simulink model "MotorImplementation"  (R2022a)
settings: Solver=FixedStepAuto  StartTime=0.0  StopTime=60  FixedStep=1/25  RelTol=1e-3
model workspace (MATLAB code in the model file):
  | %% Mechanical Parameters
  | d_Drum = 23.23e-2; % Meter
  | Drum_Friction = 0.001; % Ns/m
  | Drum_Inertia = 1.0; %kgm^2
  | 
  | n_sh = 5;
  | 
  | %% Load Case 1
  | Hs = 2.2; % m
  | T_w = 8.0; % s
  | m_payload = 8000; % kg
  | h_payload_0 = 75; % m
  | h_payload_final = h_payload_0; % m
  | h_seabed = 350; % m
  | 
  | %% Load Case 2
  | Hs = 2.2; % m
  | T_w = 8.0; % s
  | m_payload = 8000; % kg
  | h_payload_0 = 75; % m
  | h_payload_final = 15; % m
  | h_seabed = 350; % m
  | 
  | %% Load Case 3
  | Hs = 2.2; % m
  | T_w = 8.0; % s
  | m_payload = 8000; % kg
  | h_payload_0 =15; % m
  | h_payload_final = 0; % m
  | h_seabed = 350; % m
  | 
  | %% Sensors
  | % Noise simulation
  | sigma_w = 0.5; %m/s^2 (Standard deviation of noise)
  | beta = 10000; % Positive constant [-]
  | 
  | %% Payload parameters
  | % mass already defined (8000kg)
  | Volume_pl = 2; %m^3
  | Area_pl = 1.5; %m^2
  | C_D = 1.8; %[-] Drag coefficient
  | 
  | %syms rho vel
  | %F_drag = 0.5 * rho * vel^2 * C_D * Area_pl; % Density of sea water(surface) approx 1.025 kg/m^3, velocity comes from the simulation.
  | 
  | %% Seabed
  | k_spring = 1.8e6; %N/m
  | b_damper = 6.5e5; %Ns/m
  | rho = 1.025;
  | %syms delta_x
  | %if delta_x < 0
  | %    F_sb = 0;
  | %else
  | %    F_sb = k_spring*delta_x + b_damper*vel*sqrt(delta_x);
  | %end
  | 
  | %% Bouyant force
  | % The force pushing upwards when something floats down in water. Dependend
  | % on the fluid density, volume of the object falling and gravity
  | g = 9.81;
  | %F_boy = rho * Volume_pl * g;
  | 
  | %% Mechanical Parameters
  | T_N = 579 % Nominal torque [Nm]
  | PF_N = 0.85; % Nominal power factor
  | f=50;
  | n_N = 1483; % mechanical speed [rpm]
  | P_N = 90000 % Nominal mechanical power [W]
  | U = 400; % line-to-line rms stator voltage [V]
  | eta_N = 0.947; % efficiency
  | n_p = 2; % pole pairs
  | I_N=160;
  | 
  | %% Electrical parameters
  | % T-circuit
  | Rs = 0.04264;
  | L_sl = 0.3172;
  | Lm = 5.3031;
  | L_rl = 0.3172;
  | R_R = 0.0288;
  | psi_R = 20*P_N/(sqrt(2)*pi*n_p*I_N*n_N);
  | %Inv Gamma Transform
  | Lr = 5.3031 + 0.3172;
  | L_M = 5.3031^2/Lr;
  | L_M_hat = 5;
  | 
  | PSI_R = 5.3031/Lr * psi_R;
  | L_sigma =((5.3031+0.3172) - Lr);
  | %L_sigma_hat = 0.12;
  | RR = (5.3031/Lr)^2 * 0.0288;
  | %RR_Hat = 0.025;
  | R_R_opt = 0.0193;
  | X_M_opt = 2.81;
  | X_sig_opt = 0.0445;
  | 
  | R_R_hat = 0.02;
  | X_M_hat = 3;
  | X_sig_hat = 0.05;
  | R_s = 0.04264;
  | %% Control parameters
  | omega_bw = log(9)/1e-3;
  | kp = omega_bw * X_sig_hat;
  | ki = omega_bw^2 * X_sig_hat;
undefined symbols (not defined in the file): I_max, L_sigma_hat, magnitude, omega_1_N, psi_ref, R_hat, RR_Hat, Ts, V_base, w_BW
libraries: fl_lib x22, nesl_utility x10, CustomComponents_lib x6, slpidlib x4, simulink x3, eeTransforms x2, sdl_lib x1
(part 1 of 2)
settings Model: Creator=Jakob  LastModifiedBy=Jakob
settings DebuggingCC: AlgebraicLoopMsg=none

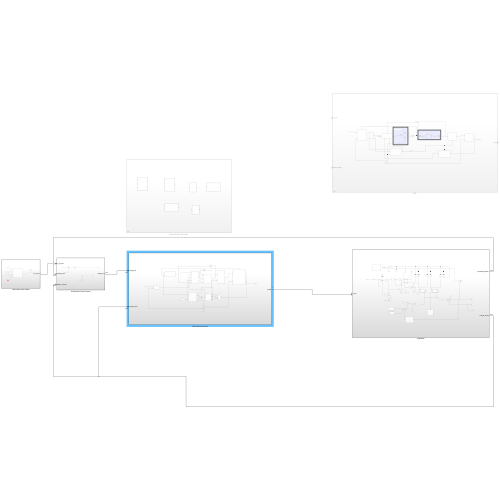
[thumbnail: Simulink's stored preview of the top-level diagram]
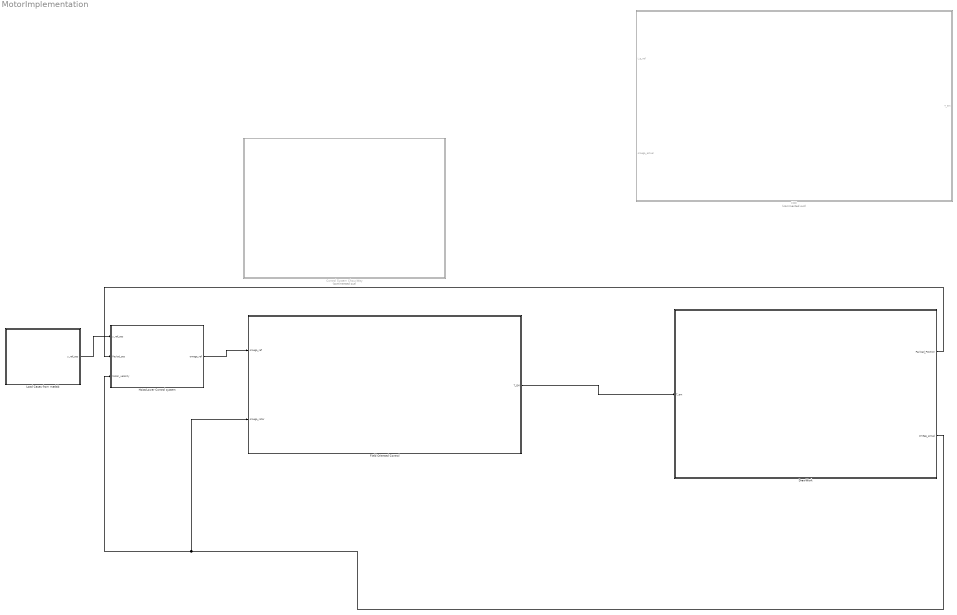
== system MotorImplementation ==
  Control System ChouxWay : Subsystem  Commented=on
  DrawWork : Subsystem
  FOC : Subsystem  Commented=on
  Field Oriented Control : Subsystem
  Hoist/Lower Control system : Subsystem
  Load Cases from matlab : Subsystem
  wires:
  Load Cases from matlab/1(y_ref_pos) -> Hoist/Lower Control system/1(y_ref_pos)
  DrawWork/1(Payload_Position) -> Hoist/Lower Control system/2(Paylod_pos)
  DrawWork/2(omega_actual) -> Field Oriented Control/2(omega_rotor), Hoist/Lower Control system/3(Motor_velocity)
  Field Oriented Control/1(T_EM) -> DrawWork/1(T_em)
  Hoist/Lower Control system/1(omega_ref) -> Field Oriented Control/1(omega_ref)

== system MotorImplementation/Control System ChouxWay ==
  Current Controller : Subsystem
  Field Weakening : Subsystem
  FluxEstimator : Subsystem
  IM Motor : Subsystem
  abc > dq : Subsystem
  "dq -> ABC" : Subsystem

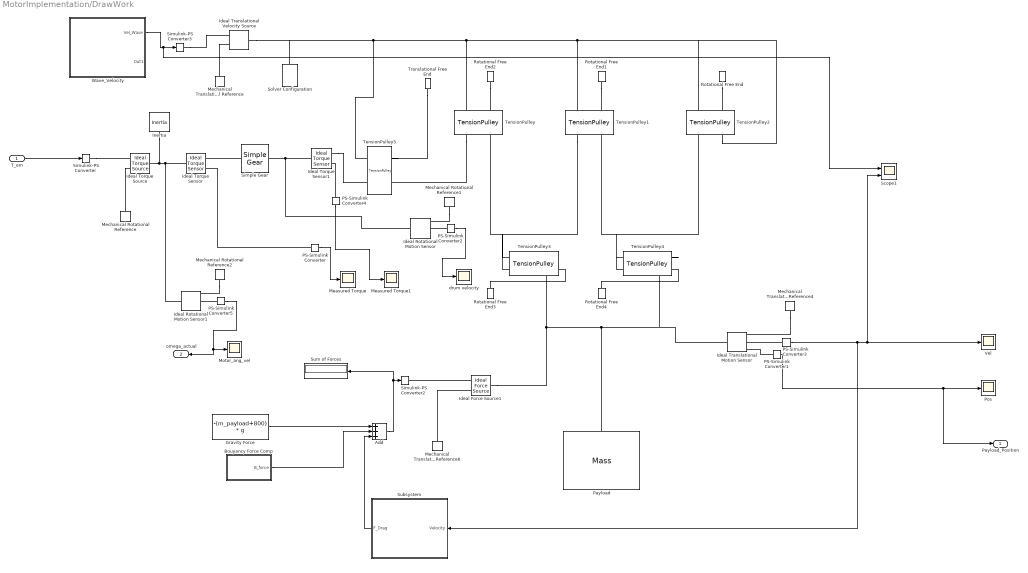
== system MotorImplementation/DrawWork ==
  T_em : Inport
  Add : Sum  Inputs=+++
  Bouyancy Force Comp : Subsystem
  Gravity Force : Constant  Value=-(m_payload+800) * g
  Ideal Force Source1 : fl_lib/Mechanical/Mechanical Sources/Ideal Force Source
      settings: SourceProductBaseCode=PW,SS,VE
  Ideal Rotational Motion Sensor : fl_lib/Mechanical/Mechanical Sensors/Ideal Rotational Motion Sensor  wrap_angle=simscape.enum.onoff.off  offset=0 rad
      settings: SourceProductBaseCode=PW,SS,VE
  Ideal Rotational Motion Sensor1 : fl_lib/Mechanical/Mechanical Sensors/Ideal Rotational Motion Sensor  wrap_angle=simscape.enum.onoff.off  offset=0 rad
      settings: SourceProductBaseCode=PW,SS,VE
  Ideal Torque Sensor : fl_lib/Mechanical/Mechanical Sensors/Ideal Torque Sensor
      settings: SourceProductBaseCode=PW,SS,VE
  Ideal Torque Sensor1 : fl_lib/Mechanical/Mechanical Sensors/Ideal Torque Sensor
      settings: SourceProductBaseCode=PW,SS,VE
  Ideal Torque Source : fl_lib/Mechanical/Mechanical Sources/Ideal Torque Source
      settings: SourceProductBaseCode=PW,SS,VE
  Ideal Translational Motion Sensor : fl_lib/Mechanical/Mechanical Sensors/Ideal Translational Motion Sensor  offset=70 m
      settings: SourceProductBaseCode=PW,SS,VE
  Ideal Translational Velocity Source : fl_lib/Mechanical/Mechanical Sources/Ideal Translational Velocity Source
      settings: SourceProductBaseCode=PW,SS,VE
  Inertia : fl_lib/Mechanical/Rotational Elements/Inertia  inertia=1.5 kg*m^2  num_ports=foundation.enum.numPorts2.one  w_specify=off  w_priority=High  w=0 rad/s  w_nominal_specify=off  w_nominal_unit=rad/s  w_nominal_value=1  t_specify=on  t_priority=None  t=500 N*m  t_nominal_specify=off  t_nominal_unit=N*m  t_nominal_value=1
      settings: SourceProductBaseCode=PW,SS,VE
  Measured Torque : Scope
  Measured Torque1 : Scope
  Mechanical Rotational Reference : fl_lib/Mechanical/Rotational Elements/Mechanical Rotational Reference
      settings: SourceProductBaseCode=PW,SS,VE
  Mechanical Rotational Reference1 : fl_lib/Mechanical/Rotational Elements/Mechanical Rotational Reference
      settings: SourceProductBaseCode=PW,SS,VE
  Mechanical Rotational Reference2 : fl_lib/Mechanical/Rotational Elements/Mechanical Rotational Reference
      settings: SourceProductBaseCode=PW,SS,VE
  Mechanical Translational Reference : fl_lib/Mechanical/Translational Elements/Mechanical Translational Reference
      settings: SourceProductBaseCode=PW,SS,VE
  Mechanical Translational Reference4 : fl_lib/Mechanical/Translational Elements/Mechanical Translational Reference
      settings: SourceProductBaseCode=PW,SS,VE
  Mechanical Translational Reference6 : fl_lib/Mechanical/Translational Elements/Mechanical Translational Reference
      settings: SourceProductBaseCode=PW,SS,VE
  Motor_ang_vel : Scope
  PS-Simulink Converter{,1..5} (6 alike) : nesl_utility/PS-Simulink Converter  PhysicalDomain=network_engine_domain  SubClassName=ps_output  LeftPortType=input  RightPortType=output  PseudoPeriodic=off  Frequencies=[]  VectorFormat=inherit  Unit=inherit  AffineConversion=off
      settings: SourceProductBaseCode=SS,PW,VE
  Payload : fl_lib/Mechanical/Translational Elements/Mass  mass=8800 kg  num_ports=foundation.enum.numPorts2.one  v_specify=off  v_priority=High  v=0 m/s  v_nominal_specify=off  v_nominal_unit=m/s  v_nominal_value=1  f_specify=off  f_priority=None  f=0 N  f_nominal_specify=off  f_nominal_unit=N  f_nominal_value=1
      settings: SourceProductBaseCode=PW,SS,VE
  Pos : Scope
  Rotational Free End{,1..4} (5 alike) : fl_lib/Mechanical/Rotational Elements/Rotational Free End  w_specify=off  w_priority=None  w=0 rad/s  w_nominal_specify=off  w_nominal_unit=rad/s  w_nominal_value=1
      settings: SourceProductBaseCode=PW,SS,VE
  Scope1 : Scope  NumInputPorts=2
  Simple Gear : sdl_lib/Gears/Simple Gear  ratio=5  rotation_direction=sdl.enum.shaftOutputDirection.opposite  friction_model=sdl.enum.gear_efficiencies_load.off  T_noload=0.1 N*m  T_nom=5 N*m  efficiency_nom=0.8  efficiency=0.8  temperature_TLU=[280, 300, 320] K  load_TLU=[1, 5, 10] N*m  efficiency_TLU=[.95, .9, .85]  efficiency_TLU2=[.85, .8, .75; .95, .9, .85; .85, .8, .7]  w_thr=0.01 rad/s  pwr_thr=0.001 W  backlash_model=sdl.enum.backlashModel.Off  backlash_distance=1e-3 mm  x0=0 mm  r_base=0.1 m  hardstop_model=simscape.enum.hardstop.smooth  transition=1e-4 mm  backlash_stiffness=1e7 N/m  backlash_damping=1e6 N*s/m  e=0  v_tol=0.001 m/s  mu_visc=[0, 0] N*m*s/rad  enable_faults=simscape.enum.onoff.off  efficiency_fault=0.05  external_fault=simscape.enum.onoff.off  temporal_fault=simscape.enum.onoff.off  fault_time=5 s  fault_angles=pi / 12 rad  report_fault=simscape.enum.assert.action.none  thermal_mass=50 J/K  temperature_specify=off  temperature_priority=High  temperature=300 K  temperature_nominal_specify=off  temperature_nominal_unit=K  temperature_nominal_value=1  x_backlash_specify=off  x_backlash_priority=None  x_backlash=0 mm  x_backlash_nominal_specify=off  x_backlash_nominal_unit=mm  x_backlash_nominal_value=1  f_hardstop_specify=off  f_hardstop_priority=None  f_hardstop=0 N  f_hardstop_nominal_specify=off  f_hardstop_nominal_unit=N  f_hardstop_nominal_value=1  v_backlash_specify=off  v_backlash_priority=None  v_backlash=0 m/s  v_backlash_nominal_specify=off  v_backlash_nominal_unit=m/s  v_backlash_nominal_value=1
  Simulink-PS Converter : nesl_utility/Simulink-PS Converter  PhysicalDomain=network_engine_domain  SubClassName=ps_input  LeftPortType=input  RightPortType=output  PseudoPeriodic=off  Frequencies=[]  NoiseDistribution=none  NoiseParameters=[]  Unit=1  AffineConversion=off  FilteringAndDerivatives=provide  SimscapeFilterOrder=1  InputFilterTimeConstant=0.001  UdotUserProvided=0
      settings: SourceProductBaseCode=SS,PW,VE
  Simulink-PS Converter2 : nesl_utility/Simulink-PS Converter  PhysicalDomain=network_engine_domain  SubClassName=ps_input  LeftPortType=input  RightPortType=output  PseudoPeriodic=off  Frequencies=[]  NoiseDistribution=none  NoiseParameters=[]  Unit=1  AffineConversion=off  FilteringAndDerivatives=provide  SimscapeFilterOrder=1  InputFilterTimeConstant=0.001  UdotUserProvided=0
      settings: SourceProductBaseCode=SS,PW,VE
  Simulink-PS Converter3 : nesl_utility/Simulink-PS Converter  PhysicalDomain=network_engine_domain  SubClassName=ps_input  LeftPortType=input  RightPortType=output  PseudoPeriodic=off  Frequencies=[]  NoiseDistribution=none  NoiseParameters=[]  Unit=1  AffineConversion=off  FilteringAndDerivatives=filter  SimscapeFilterOrder=2  InputFilterTimeConstant=0.001  UdotUserProvided=0
      settings: SourceProductBaseCode=SS,PW,VE
  Solver Configuration : nesl_utility/Solver Configuration  PhysicalDomain=network_engine_domain  SubClassName=solver  LeftPortType=input  RightPortType=generic  Tones=[]  Harmonics=[]  SimulateNoise=off  Profile=off  UseLocalSampling=off  EnableSwitchedLinearOptims=on  FrequencyDomain=off  UseCCode=off  RelTol=0.001  AbsTol=0.001  MinStep=1e-09  ToWorkspace=off  RevertToSquareIcSolve=off  NumHomotopyIterations=100  PhasorMode=off  PhasorModeNumHarmonics=1  IndexReductionMethod=DerivativeReplacement  DoDC=off  ResidualTolerance=1e-09  UseLocalSolver=off  LocalSolverChoice=NE_BACKWARD_EULER_ADVANCER  LocalSolverSampleTime=0.001  DoFixedCost=off  MaxNonlinIter=3  MaxModeIter=2  ComputeImpulses=off  ImpulseIterations=2  LinearAlgebra=auto  LinearAlgebraNumThread=0  EquationFormulation=NE_TIME_EF  DelaysMemoryBudget=1024  AutomaticFiltering=on  FilteringTimeConstant=0.001  PartitionStorageMethod=AS_NEEDED  PartitionMemoryBudget=1024  PartitionMethod=ROBUST
      settings: SourceProductBaseCode=SS,PW,VE
  Subsystem : Subsystem
  Sum of Forces : Display
  TensionPulley{,1..2,4} (4 alike) : CustomComponents_lib/TensionPulley  radius=0.1 m  b_damp=0 N*m*s/rad  inertia=0.00001 kg*m^2  mass=0.1 kg  mu_s=1  f_A_specify=off  f_A_priority=None  f_A=0 N  f_A_nominal_specify=off  f_A_nominal_unit=N  f_A_nominal_value=1  f_B_specify=off  f_B_priority=None  f_B=0 N  f_B_nominal_specify=off  f_B_nominal_unit=N  f_B_nominal_value=1  f_C_specify=off  f_C_priority=None  f_C=0 N  f_C_nominal_specify=off  f_C_nominal_unit=N  f_C_nominal_value=1  tau_specify=off  tau_priority=None  tau=0 N*m  tau_nominal_specify=off  tau_nominal_unit=N*m  tau_nominal_value=1  w_specify=off  w_priority=None  w=0 rad/s  w_nominal_specify=off  w_nominal_unit=rad/s  w_nominal_value=1  v_specify=off  v_priority=None  v=0 m/s  v_nominal_specify=off  v_nominal_unit=m/s  v_nominal_value=1
      settings: InternalSimscapePortConfiguration="{\"Bottom\":[],\"Left\":[{\"id\":\"C\",\"label\":\"C\",\"type\":\"foundation.mechanical.translational.translational\"},{\"id\":\"S\",\"label\":\"S\",\"type\":\"foundation.mechanical.rotational.rotational\"}],\"Right\":[{\"id\":\"A\",\"label\":\"A\",\"type\":\"foundation.mechanical.translational.translational\"},{\"id\":\"B\",\"label\":\"B\",\"type\":\"foundation.mechanical.translational.translational\"}],\"Top\":[]}"
  TensionPulley3 : CustomComponents_lib/TensionPulley  radius=0.1 m  b_damp=0 N*m*s/rad  inertia=00.00001 kg*m^2  mass=0.1 kg  mu_s=1  f_A_specify=off  f_A_priority=None  f_A=0 N  f_A_nominal_specify=off  f_A_nominal_unit=N  f_A_nominal_value=1  f_B_specify=off  f_B_priority=None  f_B=0 N  f_B_nominal_specify=off  f_B_nominal_unit=N  f_B_nominal_value=1  f_C_specify=off  f_C_priority=None  f_C=0 N  f_C_nominal_specify=off  f_C_nominal_unit=N  f_C_nominal_value=1  tau_specify=off  tau_priority=None  tau=0 N*m  tau_nominal_specify=off  tau_nominal_unit=N*m  tau_nominal_value=1  w_specify=off  w_priority=None  w=0 rad/s  w_nominal_specify=off  w_nominal_unit=rad/s  w_nominal_value=1  v_specify=off  v_priority=None  v=0 m/s  v_nominal_specify=off  v_nominal_unit=m/s  v_nominal_value=1
      settings: InternalSimscapePortConfiguration="{\"Bottom\":[],\"Left\":[{\"id\":\"C\",\"label\":\"C\",\"type\":\"foundation.mechanical.translational.translational\"},{\"id\":\"S\",\"label\":\"S\",\"type\":\"foundation.mechanical.rotational.rotational\"}],\"Right\":[{\"id\":\"A\",\"label\":\"A\",\"type\":\"foundation.mechanical.translational.translational\"},{\"id\":\"B\",\"label\":\"B\",\"type\":\"foundation.mechanical.translational.translational\"}],\"Top\":[]}"
  TensionPulley5 : CustomComponents_lib/TensionPulley  radius=d_Drum/2 m  b_damp=Drum_Friction N*m*s/rad  inertia=Drum_Inertia kg*m^2  mass=0.1 kg  mu_s=1  f_A_specify=off  f_A_priority=None  f_A=0 N  f_A_nominal_specify=off  f_A_nominal_unit=N  f_A_nominal_value=1  f_B_specify=off  f_B_priority=None  f_B=0 N  f_B_nominal_specify=off  f_B_nominal_unit=N  f_B_nominal_value=1  f_C_specify=off  f_C_priority=None  f_C=0 N  f_C_nominal_specify=off  f_C_nominal_unit=N  f_C_nominal_value=1  tau_specify=off  tau_priority=None  tau=0 N*m  tau_nominal_specify=off  tau_nominal_unit=N*m  tau_nominal_value=1  w_specify=off  w_priority=None  w=0 rad/s  w_nominal_specify=off  w_nominal_unit=rad/s  w_nominal_value=1  v_specify=off  v_priority=None  v=0 m/s  v_nominal_specify=off  v_nominal_unit=m/s  v_nominal_value=1
      settings: InternalSimscapePortConfiguration="{\"Bottom\":[],\"Left\":[{\"id\":\"C\",\"label\":\"C\",\"type\":\"foundation.mechanical.translational.translational\"},{\"id\":\"S\",\"label\":\"S\",\"type\":\"foundation.mechanical.rotational.rotational\"}],\"Right\":[{\"id\":\"A\",\"label\":\"A\",\"type\":\"foundation.mechanical.translational.translational\"},{\"id\":\"B\",\"label\":\"B\",\"type\":\"foundation.mechanical.translational.translational\"}],\"Top\":[]}"
  Translational Free End : fl_lib/Mechanical/Translational Elements/Translational Free End  v_specify=off  v_priority=None  v=0 m/s  v_nominal_specify=off  v_nominal_unit=m/s  v_nominal_value=1
      settings: SourceProductBaseCode=PW,SS,VE  InternalSimscapePortConfiguration="{\"Bottom\":[],\"Left\":[{\"id\":\"V\",\"label\":\"\",\"type\":\"foundation.mechanical.translational.translational\"}],\"Right\":[],\"Top\":[]}"
  Vel : Scope
  Wave_Velocity : Subsystem
  drum velocity : Scope
  Payload_Position : Outport
  omega_actual : Outport  Port=2
  wires:
  Subsystem/1(F_Drag) -> Add/3
  Bouyancy Force Comp/1(B_force) -> Add/2
  Add/1 -> Sum of Forces/1, Simulink-PS Converter2/1
  PS-Simulink Converter2/1 -> drum velocity/1
  PS-Simulink Converter/1 -> Measured Torque/1
  Wave_Velocity/1(Vel_Wave) -> Scope1/1, Simulink-PS Converter3/1
  PS-Simulink Converter3/1 -> Subsystem/1(Velocity), Scope1/2, Vel/1
  Gravity Force/1 -> Add/1
  PS-Simulink Converter1/1 -> Payload_Position/1, Pos/1
  PS-Simulink Converter4/1 -> Measured Torque1/1
  PS-Simulink Converter5/1 -> omega_actual/1, Motor_ang_vel/1
  T_em/1 -> Simulink-PS Converter/1
  connections:
  Ideal Torque Source/LConn1 -- Inertia/LConn1 -- Ideal Rotational Motion Sensor1/LConn1 -- Ideal Torque Sensor/LConn1
  TensionPulley4/LConn1 -- Ideal Translational Motion Sensor/LConn1 -- Payload/LConn1 -- TensionPulley3/LConn1 -- Ideal Force Source1/LConn1
  TensionPulley/LConn1 -- TensionPulley2/LConn1 -- TensionPulley2/RConn2 -- TensionPulley1/LConn1 -- TensionPulley5/LConn1 -- Solver Configuration/RConn1 -- Ideal Translational Velocity Source/LConn1
  Rotational Free End3/LConn1 -- TensionPulley3/LConn2
  TensionPulley4/RConn1 -- TensionPulley2/RConn1
  Simulink-PS Converter/RConn1 -- Ideal Torque Source/RConn1
  Ideal Force Source1/RConn1 -- Simulink-PS Converter2/RConn1
  Rotational Free End/LConn1 -- TensionPulley2/LConn2
  Mechanical Rotational Reference1/LConn1 -- Ideal Rotational Motion Sensor/RConn1
  Simulink-PS Converter3/RConn1 -- Ideal Translational Velocity Source/RConn1
  PS-Simulink Converter1/LConn1 -- Ideal Translational Motion Sensor/RConn3
  PS-Simulink Converter2/LConn1 -- Ideal Rotational Motion Sensor/RConn2
  Mechanical Rotational Reference/LConn1 -- Ideal Torque Source/RConn2
  Mechanical Translational Reference6/LConn1 -- Ideal Force Source1/RConn2
  Ideal Rotational Motion Sensor/LConn1 -- Simple Gear/RConn1 -- Ideal Torque Sensor1/LConn1
  Rotational Free End4/LConn1 -- TensionPulley4/LConn2
  PS-Simulink Converter3/LConn1 -- Ideal Translational Motion Sensor/RConn2
  TensionPulley3/RConn2 -- TensionPulley/RConn2
  TensionPulley4/RConn2 -- TensionPulley1/RConn2
  Mechanical Translational Reference4/LConn1 -- Ideal Translational Motion Sensor/RConn1
  PS-Simulink Converter/LConn1 -- Ideal Torque Sensor/RConn2
  Rotational Free End1/LConn1 -- TensionPulley1/LConn2
  TensionPulley1/RConn1 -- TensionPulley3/RConn1
  Mechanical Translational Reference/LConn1 -- Ideal Translational Velocity Source/RConn2
  Rotational Free End2/LConn1 -- TensionPulley/LConn2
  TensionPulley/RConn1 -- TensionPulley5/RConn2
  Translational Free End/LConn1 -- TensionPulley5/RConn1
  Ideal Torque Sensor1/RConn1 -- TensionPulley5/LConn2
  PS-Simulink Converter4/LConn1 -- Ideal Torque Sensor1/RConn2
  Simple Gear/LConn1 -- Ideal Torque Sensor/RConn1
  PS-Simulink Converter5/LConn1 -- Ideal Rotational Motion Sensor1/RConn2
  Mechanical Rotational Reference2/LConn1 -- Ideal Rotational Motion Sensor1/RConn1

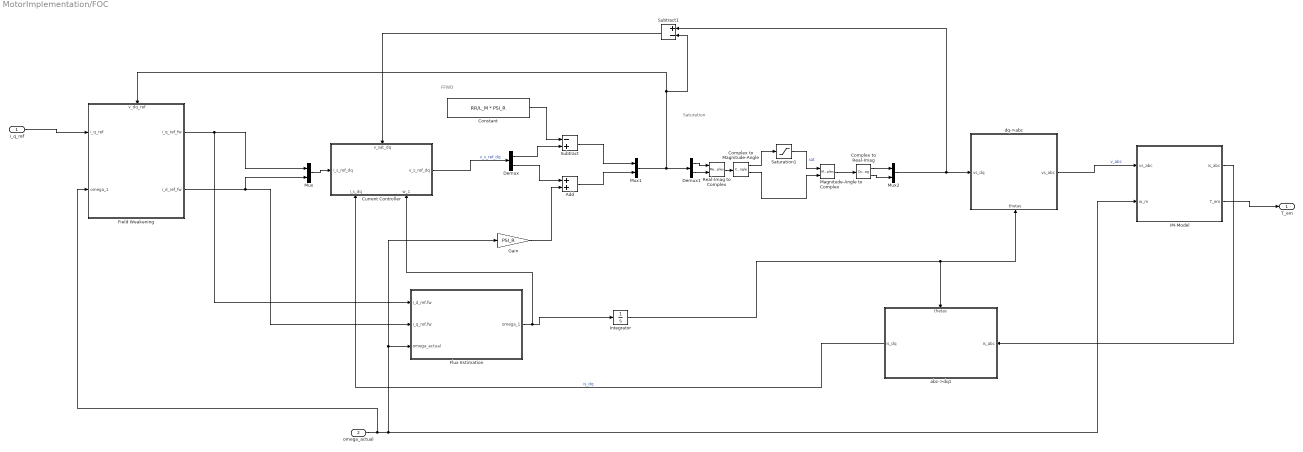
== system MotorImplementation/FOC ==
  note: Saturation
  note: FFWD
  i_q_ref : Inport
  omega_actual : Inport  Port=2
  Add : Sum
  Complex to Magnitude-Angle : ComplexToMagnitudeAngle
  Complex to Real-Imag : ComplexToRealImag
  Constant : Constant  Value=RR/L_M * PSI_R
  Current Controller : Subsystem
      settings: PortSchema="{\"entries\":[{\"content\":{\"sides\":[{\"content\":{\"connectorIds\":[\"In1\"]},\"type\":\"ConnectorPlacement.EquallySpacedRectSide\",\"uuid\":\"97c548b6-6990-4323-a853-1e64e742285c\"},{\"content\":{\"connectorIds\":[\"Out1\"],\"side\":\"RIGHT\"},\"type\":\"ConnectorPlacement.EquallySpacedRectSide\",\"uuid\":\"cacb7644-0a67-4de4-9bb2-887734fe331a\"},{\"content\":{\"connectorIds\":[\"In2\"],\"side\":\"TOP\"},\"type\":\"ConnectorPlacement.EquallySpacedRectSide\",\"uuid\":\"a20c1423-7334-426c-a525-8bdb26886bc3\"},{\"content\":{\"connectorIds\":[\"In3\",\"In4\"],\"side\":\"BOTTOM\"},\"type\":\"ConnectorPlacement.EquallySpacedRectSide\",\"uuid\":\"b9821709-22a3-4c1b-ad46-11760bdb190f\"}]},\"type\":\"ConnectorPlacement.EquallySpacedConnector\",\"uuid\":\"74caaff1-86aa-4f34-8e3a-31d84a5552f1\"}],\"packageUris\":[\"http://schema.mathworks.com/mf0/Connector/R2020b\"],\"version\":\"1.0\"}"
  Demux : Demux  Outputs=2
  Demux1 : Demux  Outputs=2
  Field Weakening : Subsystem
      settings: PortSchema="{\"entries\":[{\"content\":{\"sides\":[{\"content\":{\"connectorIds\":[\"In1\",\"In2\"]},\"type\":\"ConnectorPlacement.EquallySpacedRectSide\",\"uuid\":\"92991972-79b1-4c20-b1be-c048af0edf88\"},{\"content\":{\"connectorIds\":[\"Out1\",\"Out2\"],\"side\":\"RIGHT\"},\"type\":\"ConnectorPlacement.EquallySpacedRectSide\",\"uuid\":\"cfb4a663-faee-454f-9ec9-68645b776424\"},{\"content\":{\"connectorIds\":[\"In3\"],\"side\":\"TOP\"},\"type\":\"ConnectorPlacement.EquallySpacedRectSide\",\"uuid\":\"6b878172-644f-4a73-b905-9ff1fa4855ef\"}]},\"type\":\"ConnectorPlacement.EquallySpacedConnector\",\"uuid\":\"11cec5aa-34fb-4a6f-afd2-d847060dc809\"}],\"packageUris\":[\"http://schema.mathworks.com/mf0/Connector/R2020b\"],\"version\":\"1.0\"}"
  Flux Estimation : Subsystem
  Gain : Gain  Gain=PSI_R
  IM-Model : Subsystem
  Integrator : Integrator
  Magnitude-Angle to Complex : MagnitudeAngleToComplex
  Mux : Mux  Inputs=2
  Mux1 : Mux  Inputs=2
  Mux2 : Mux  Inputs=2
  Real-Imag to Complex : RealImagToComplex
  Saturation1 : Saturate  UpperLimit=400*sqrt(2)/sqrt(3)
  Subtract : Sum  Inputs=-+
  Subtract1 : Sum  Inputs=+-
  abc->dq1 : Subsystem
      settings: PortSchema="{\"entries\":[{\"content\":{\"sides\":[{\"content\":{\"connectorIds\":[\"In1\"]},\"type\":\"ConnectorPlacement.EquallySpacedRectSide\",\"uuid\":\"c3863cce-4a98-427c-9e63-89298f679a84\"},{\"content\":{\"connectorIds\":[\"Out1\"],\"side\":\"RIGHT\"},\"type\":\"ConnectorPlacement.EquallySpacedRectSide\",\"uuid\":\"ae3c4991-ab62-4114-9bee-e9a7348a29ce\"},{\"content\":{\"connectorIds\":[\"In2\"],\"side\":\"TOP\"},\"type\":\"ConnectorPlacement.EquallySpacedRectSide\",\"uuid\":\"fea582b6-68e0-450b-8231-0f2cf258215e\"},{\"content\":{\"connectorIds\":[],\"side\":\"BOTTOM\"},\"type\":\"ConnectorPlacement.EquallySpacedRectSide\",\"uuid\":\"4cb5cb50-d1c5-41cc-b580-d3f7a61a133b\"}]},\"type\":\"ConnectorPlacement.EquallySpacedConnector\",\"uuid\":\"936995e1-3667-4d5a-83ac-5ed23eb7cec5\"}],\"packageUris\":[\"http://schema.mathworks.com/mf0/Connector/R2020b\"],\"version\":\"1.0\"}"
  dq->abc : Subsystem
      settings: PortSchema="{\"entries\":[{\"content\":{\"sides\":[{\"content\":{\"connectorIds\":[\"In1\"]},\"type\":\"ConnectorPlacement.EquallySpacedRectSide\",\"uuid\":\"c3863cce-4a98-427c-9e63-89298f679a84\"},{\"content\":{\"connectorIds\":[\"Out1\"],\"side\":\"RIGHT\"},\"type\":\"ConnectorPlacement.EquallySpacedRectSide\",\"uuid\":\"ae3c4991-ab62-4114-9bee-e9a7348a29ce\"},{\"content\":{\"connectorIds\":[],\"side\":\"TOP\"},\"type\":\"ConnectorPlacement.EquallySpacedRectSide\",\"uuid\":\"fea582b6-68e0-450b-8231-0f2cf258215e\"},{\"content\":{\"connectorIds\":[\"In2\"],\"side\":\"BOTTOM\"},\"type\":\"ConnectorPlacement.EquallySpacedRectSide\",\"uuid\":\"09df17c4-38be-4fcd-b44b-abaf9d5b2651\"}]},\"type\":\"ConnectorPlacement.EquallySpacedConnector\",\"uuid\":\"936995e1-3667-4d5a-83ac-5ed23eb7cec5\"}],\"packageUris\":[\"http://schema.mathworks.com/mf0/Connector/R2020b\"],\"version\":\"1.0\"}"
  T_em : Outport
  wires:
  Flux Estimation/1(omega_1) -> Current Controller/4(w_1), Integrator/1
  Field Weakening/1(i_q_ref_fw) -> Mux/1, Flux Estimation/1(i_d_ref.fw)
  omega_actual/1 -> IM-Model/2(w_m), Gain/1, Flux Estimation/3(omega_actual), Field Weakening/2(omega_1)
  i_q_ref/1 -> Field Weakening/1(i_q_ref)
  Field Weakening/2(i_d_ref_fw) -> Flux Estimation/2(i_q_ref.fw), Mux/2
  Mux/1 -> Current Controller/1(i_s_ref_dq)
  Current Controller/1(v_s_ref_dq) -> Demux/1  "v_s_ref_dq"
  Gain/1 -> Add/2
  Constant/1 -> Subtract/1
  Demux/1 -> Subtract/2
  Demux/2 -> Add/1
  Subtract/1 -> Mux1/1
  Add/1 -> Mux1/2
  Demux1/2 -> Real-Imag to Complex/2
  Mux2/1 -> Subtract1/1, dq->abc/1(vs_dq)
  Saturation1/1 -> Magnitude-Angle to Complex/1  "sat"
  Complex to Real-Imag/2 -> Mux2/2
  Magnitude-Angle to Complex/1 -> Complex to Real-Imag/1
  Complex to Magnitude-Angle/2 -> Magnitude-Angle to Complex/2
  Mux1/1 -> Subtract1/2, Field Weakening/3(v_dq_ref), Demux1/1
  Real-Imag to Complex/1 -> Complex to Magnitude-Angle/1
  Complex to Magnitude-Angle/1 -> Saturation1/1
  Demux1/1 -> Real-Imag to Complex/1
  Complex to Real-Imag/1 -> Mux2/1
  dq->abc/1(vs_abc) -> IM-Model/1(vs_abc)  "v_abc"
  IM-Model/2(T_em) -> T_em/1
  IM-Model/1(is_abc) -> abc->dq1/1(is_abc)
  Integrator/1 -> abc->dq1/2(thetas), dq->abc/2(thetas)
  abc->dq1/1(is_dq) -> Current Controller/3(i_s_dq)  "is_dq"
  Subtract1/1 -> Current Controller/2(v_sat_dq)

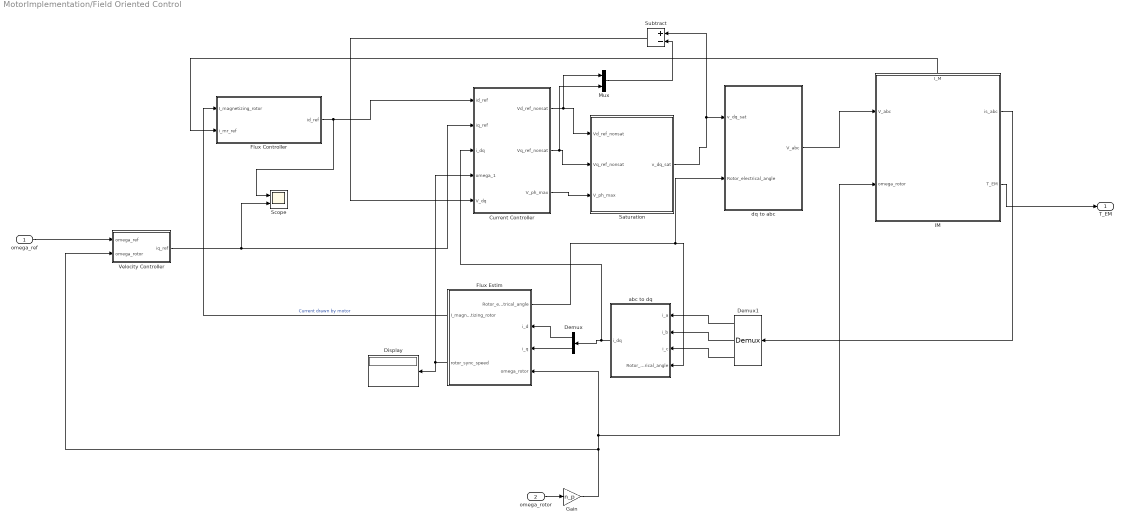
== system MotorImplementation/Field Oriented Control ==
  omega_ref : Inport
  omega_rotor : Inport  Port=2
  Current Controller : Subsystem
  Demux : Demux  Outputs=2
  Demux1 : Demux  Outputs=3
  Display : Display
  Flux Controller : Subsystem
  Flux Estim : Subsystem
      settings: PortSchema="{\"entries\":[{\"content\":{\"sides\":[{\"content\":{\"connectorIds\":[\"Out3\",\"In1\",\"In2\",\"In3\"]},\"type\":\"ConnectorPlacement.EquallySpacedRectSide\",\"uuid\":\"02f27d2e-38fe-43c2-a712-ecf44442955b\"},{\"content\":{\"connectorIds\":[\"Out1\",\"Out2\"],\"side\":\"RIGHT\"},\"type\":\"ConnectorPlacement.EquallySpacedRectSide\",\"uuid\":\"b981552c-3f2f-4bf0-a84a-f70a19a52168\"},{\"content\":{\"connectorIds\":[],\"side\":\"TOP\"},\"type\":\"ConnectorPlacement.EquallySpacedRectSide\",\"uuid\":\"d3509bb5-0c97-45b5-b720-2a84b0add849\"}]},\"type\":\"ConnectorPlacement.EquallySpacedConnector\",\"uuid\":\"e3c2788d-83db-462b-b1be-711107b53b95\"}],\"packageUris\":[\"http://schema.mathworks.com/mf0/Connector/R2020b\"],\"version\":\"1.0\"}"
  Gain : Gain  Gain=n_p
  IM : Subsystem
      settings: PortSchema="{\"entries\":[{\"content\":{\"sides\":[{\"content\":{\"connectorIds\":[\"In1\",\"In2\"]},\"type\":\"ConnectorPlacement.EquallySpacedRectSide\",\"uuid\":\"087ae8eb-b8c6-4f38-a1ca-e2f592f510df\"},{\"content\":{\"connectorIds\":[\"Out1\",\"Out2\"],\"side\":\"RIGHT\"},\"type\":\"ConnectorPlacement.EquallySpacedRectSide\",\"uuid\":\"93b8f370-135e-4e29-a4a2-dbfa81101af4\"},{\"content\":{\"connectorIds\":[\"Out3\"],\"side\":\"TOP\"},\"type\":\"ConnectorPlacement.EquallySpacedRectSide\",\"uuid\":\"461b04e0-7865-43b9-aa58-881bc3ba1c85\"}]},\"type\":\"ConnectorPlacement.EquallySpacedConnector\",\"uuid\":\"579e4038-afa0-4a6a-ac23-27775a3ef245\"}],\"packageUris\":[\"http://schema.mathworks.com/mf0/Connector/R2020b\"],\"version\":\"1.0\"}"
  Mux : Mux  Inputs=2
  Saturation : Subsystem
  Scope : Scope  NumInputPorts=2
  Subtract : Sum  Inputs=+-
  Velocity Controller : Subsystem
  abc to dq : Subsystem
  dq to abc : Subsystem
  T_EM : Outport
  wires:
  IM/3(I_M) -> Flux Controller/2(i_mr_ref)
  dq to abc/1(V_abc) -> IM/1(V_abc)
  Velocity Controller/1(iq_ref) -> Scope/2, Current Controller/2(iq_ref)
  omega_rotor/1 -> Gain/1
  omega_ref/1 -> Velocity Controller/1(omega_ref)
  Mux/1 -> Subtract/2
  Demux1/1 -> abc to dq/1(i_a)
  Current Controller/2(Vq_ref_nonsat) -> Mux/2, Saturation/2(Vq_ref_nonsat)
  Flux Estim/1(I_magnetizing_rotor) -> Flux Controller/1(I_magnetizing_rotor)  "Current drawn by motor"
  Flux Controller/1(id_ref) -> Scope/1, Current Controller/1(id_ref)
  Saturation/1(v_dq_sat) -> Subtract/1, dq to abc/1(v_dq_sat)
  Flux Estim/2(rotor_sync_speed) -> Current Controller/4(omega_1), Display/1
  Demux1/2 -> abc to dq/2(i_b)
  IM/1(is_abc) -> Demux1/1
  Demux1/3 -> abc to dq/3(i_c)
  Subtract/1 -> Current Controller/5(V_dq)
  Demux/2 -> Flux Estim/2(i_q)
  Current Controller/1(Vd_ref_nonsat) -> Mux/1, Saturation/1(Vd_ref_nonsat)
  abc to dq/1(i_dq) -> Current Controller/3(i_dq), Demux/1
  Current Controller/3(V_ph_max) -> Saturation/3(V_ph_max)
  Flux Estim/3(Rotor_electrical_angle) -> dq to abc/2(Rotor_electrical_angle), abc to dq/4(Rotor_electrical_angle)
  Demux/1 -> Flux Estim/1(i_d)
  IM/2(T_EM) -> T_EM/1
  Gain/1 -> Velocity Controller/2(omega_rotor), IM/2(omega_rotor), Flux Estim/3(omega_rotor)

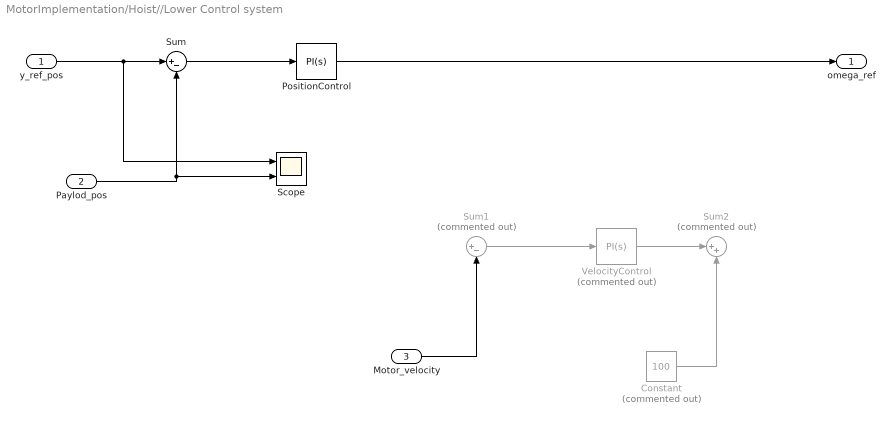
== system MotorImplementation/Hoist//Lower Control system ==
  y_ref_pos : Inport
  Paylod_pos : Inport  Port=2
  Motor_velocity : Inport  Port=3
  Constant : Constant  Commented=on  Value=100
  PositionControl : slpidlib/PID Controller  Controller=PI  Form=Parallel  TimeDomain=Continuous-time  UseExternalTs=off  SampleTime=-1  IntegratorMethod=Forward Euler  FilterMethod=Forward Euler  ControllerParametersSource=internal  P=1  I=1  UseKiTs=off  D=0  N=100  UseFilter=on  TunerSelectOption=Transfer Function Based (PID Tuner App)  InitialConditionSource=internal  InitialConditionForIntegrator=0  InitialConditionForFilter=0  DifferentiatorICPrevScaledInput=0  ExternalReset=none  TrackingMode=off  Kt=1  LimitOutput=off  SatLimitsSource=internal  UpperSaturationLimit=inf  LowerSaturationLimit=-inf  LinearizeAsGain=on  AntiWindupMode=none  Kb=1  POutMin=[]  POutMax=[]  IOutMin=[]  IOutMax=[]  DOutMin=[]  DOutMax=[]  NOutMin=[]  NOutMax=[]  SumOutMin=[]  SumOutMax=[]  SaturationOutMin=[]  SaturationOutMax=[]  PParamMin=[]  PParamMax=[]  IParamMin=[]  IParamMax=[]  DParamMin=[]  DParamMax=[]  NParamMin=[]  NParamMax=[]  KbParamMin=[]  KbParamMax=[]  KtParamMin=[]  KtParamMax=[]  KbOutMin=[]  KbOutMax=[]  KtOutMin=[]  KtOutMax=[]  IntegratorOutMin=[]  IntegratorOutMax=[]  FilterOutMin=[]  FilterOutMax=[]  SumI1OutMin=[]  SumI1OutMax=[]  SumI2OutMin=[]  SumI2OutMax=[]  SumI3OutMin=[]  SumI3OutMax=[]  SumI4OutMin=[]  SumI4OutMax=[]  SumDOutMin=[]  SumDOutMax=[]  DifferentiatorOutMin=[]  DifferentiatorOutMax=[]  FilterDiffOutCoefMin=[]  FilterDiffOutCoefMax=[]  ReciprocalOutMin=[]  ReciprocalOutMax=[]  SumDenOutMin=[]  SumDenOutMax=[]  SumNumOutMin=[]  SumNumOutMax=[]  DivideOutMin=[]  DivideOutMax=[]  UdiffTsProdOutMin=[]  UdiffTsProdOutMax=[]  NTsProdOutMin=[]  NTsProdOutMax=[]  UintegralTsProdOutMin=[]  UintegralTsProdOutMax=[]  UngainTsProdOutMin=[]  UngainTsProdOutMax=[]  IntegratorContinuousStateAttributes=''  IntegratorStateMustResolveToSignalObject=off  IntegratorRTWStateStorageClass=Auto  FilterContinuousStateAttributes=''  FilterStateMustResolveToSignalObject=off  FilterRTWStateStorageClass=Auto  ParallelPVariant=InternalParameters  IdealPVariant=Disabled  IVariant=InternalParameters  DVariant=Disabled  IntegratorVariant=Continuous  SatVariant=Disabled  AWVariant=Passthrough  PCopyVariant=Disabled  TRVariant=Disabled  FdbkBlocksVariant=Forward  IdealPFdbkVariant=Disabled  SatFdbkVariant=Disabled  DerivativeFilterVariant=Disabled  NVariant=Disabled  NCopyVariant=Disabled_SignalSpec  FilterICVariant=Disabled  IntegratorICVariant=InternalICs  ExternalResetVariant=Disabled  TRSumVariant=Passthrough  SumFdbkVariant=Disabled  SumVariant=Sum_PI  TsampFilterVariant=InternalTs  TsampNgainVariant=Passthrough  TsampIntegralVariant=Passthrough  ExternalSaturationOutDataTypeStr=Inherit: Same as second input  aMode=0
  Scope : Scope  NumInputPorts=2
  Sum : Sum  Inputs=|+-
  Sum1 : Sum  Commented=on  Inputs=|+-
  Sum2 : Sum  Commented=on  Inputs=|++
  VelocityControl : slpidlib/PID Controller  Commented=on  Controller=PI  Form=Parallel  TimeDomain=Continuous-time  UseExternalTs=off  SampleTime=-1  IntegratorMethod=Forward Euler  FilterMethod=Forward Euler  ControllerParametersSource=internal  P=1  I=1  UseKiTs=off  D=0  N=100  UseFilter=on  TunerSelectOption=Transfer Function Based (PID Tuner App)  InitialConditionSource=internal  InitialConditionForIntegrator=0  InitialConditionForFilter=0  DifferentiatorICPrevScaledInput=0  ExternalReset=none  TrackingMode=off  Kt=1  LimitOutput=off  SatLimitsSource=internal  UpperSaturationLimit=inf  LowerSaturationLimit=-inf  LinearizeAsGain=on  AntiWindupMode=none  Kb=1  POutMin=[]  POutMax=[]  IOutMin=[]  IOutMax=[]  DOutMin=[]  DOutMax=[]  NOutMin=[]  NOutMax=[]  SumOutMin=[]  SumOutMax=[]  SaturationOutMin=[]  SaturationOutMax=[]  PParamMin=[]  PParamMax=[]  IParamMin=[]  IParamMax=[]  DParamMin=[]  DParamMax=[]  NParamMin=[]  NParamMax=[]  KbParamMin=[]  KbParamMax=[]  KtParamMin=[]  KtParamMax=[]  KbOutMin=[]  KbOutMax=[]  KtOutMin=[]  KtOutMax=[]  IntegratorOutMin=[]  IntegratorOutMax=[]  FilterOutMin=[]  FilterOutMax=[]  SumI1OutMin=[]  SumI1OutMax=[]  SumI2OutMin=[]  SumI2OutMax=[]  SumI3OutMin=[]  SumI3OutMax=[]  SumI4OutMin=[]  SumI4OutMax=[]  SumDOutMin=[]  SumDOutMax=[]  DifferentiatorOutMin=[]  DifferentiatorOutMax=[]  FilterDiffOutCoefMin=[]  FilterDiffOutCoefMax=[]  ReciprocalOutMin=[]  ReciprocalOutMax=[]  SumDenOutMin=[]  SumDenOutMax=[]  SumNumOutMin=[]  SumNumOutMax=[]  DivideOutMin=[]  DivideOutMax=[]  UdiffTsProdOutMin=[]  UdiffTsProdOutMax=[]  NTsProdOutMin=[]  NTsProdOutMax=[]  UintegralTsProdOutMin=[]  UintegralTsProdOutMax=[]  UngainTsProdOutMin=[]  UngainTsProdOutMax=[]  IntegratorContinuousStateAttributes=''  IntegratorStateMustResolveToSignalObject=off  IntegratorRTWStateStorageClass=Auto  FilterContinuousStateAttributes=''  FilterStateMustResolveToSignalObject=off  FilterRTWStateStorageClass=Auto  ParallelPVariant=InternalParameters  IdealPVariant=Disabled  IVariant=InternalParameters  DVariant=Disabled  IntegratorVariant=Continuous  SatVariant=Disabled  AWVariant=Passthrough  PCopyVariant=Disabled  TRVariant=Disabled  FdbkBlocksVariant=Forward  IdealPFdbkVariant=Disabled  SatFdbkVariant=Disabled  DerivativeFilterVariant=Disabled  NVariant=Disabled  NCopyVariant=Disabled_SignalSpec  FilterICVariant=Disabled  IntegratorICVariant=InternalICs  ExternalResetVariant=Disabled  TRSumVariant=Passthrough  SumFdbkVariant=Disabled  SumVariant=Sum_PI  TsampFilterVariant=InternalTs  TsampNgainVariant=Passthrough  TsampIntegralVariant=Passthrough  ExternalSaturationOutDataTypeStr=Inherit: Same as second input  aMode=0
  omega_ref : Outport
  wires:
  y_ref_pos/1 -> Scope/1, Sum/1
  Sum/1 -> PositionControl/1
  Sum1/1 -> VelocityControl/1
  Paylod_pos/1 -> Sum/2, Scope/2
  Motor_velocity/1 -> Sum1/2
  VelocityControl/1 -> Sum2/1
  PositionControl/1 -> omega_ref/1
  Constant/1 -> Sum2/2

== system MotorImplementation/Load Cases from matlab ==
  Case Selector : MATLAB Function  TreatAsAtomicUnit=on
  Constant : Constant
  Ramp : simulink/Sources/Ramp  slope=-2.5  start=0  InitialOutput=75
  Ramp1 : simulink/Sources/Ramp  slope=-1  start=0  InitialOutput=15
  Saturation : Saturate  UpperLimit=75  LowerLimit=15
  Saturation1 : Saturate  UpperLimit=15  LowerLimit=0
  Scope : Scope
  y_ref : Constant  Value=75
  y_ref_pos : Outport
  wires:
  Case Selector/1(payload_ref_pos) -> Scope/1, y_ref_pos/1
  Constant/1 -> Case Selector/4(CaseSelector)
  y_ref/1 -> Case Selector/1(Case1)
  Ramp/1 -> Saturation/1
  Saturation/1 -> Case Selector/2(Case2)
  Ramp1/1 -> Saturation1/1
  Saturation1/1 -> Case Selector/3(Case3)

== system MotorImplementation/Control System ChouxWay/Current Controller ==
  i_s_ref_dq : Inport
  v_sat_dq : Inport  Port=2
  i_s_dq : Inport  Port=3
  w_1 : Inport  Port=4
  MATLAB Function : MATLAB Function  TreatAsAtomicUnit=on
  Unit Delay : UnitDelay  SampleTime=-1  HasFrameUpgradeWarning=on
  v_s_ref_dq : Outport  PortDimensions=2
  wires:
  v_sat_dq/1 -> MATLAB Function/1(v_sat_dq)
  Unit Delay/1 -> MATLAB Function/5(I)
  i_s_ref_dq/1 -> MATLAB Function/2(i_s_ref)
  i_s_dq/1 -> MATLAB Function/3(i_s)
  MATLAB Function/2(Inew) -> Unit Delay/1
  w_1/1 -> MATLAB Function/4(w_1)
  MATLAB Function/1(v_s_ref) -> v_s_ref_dq/1

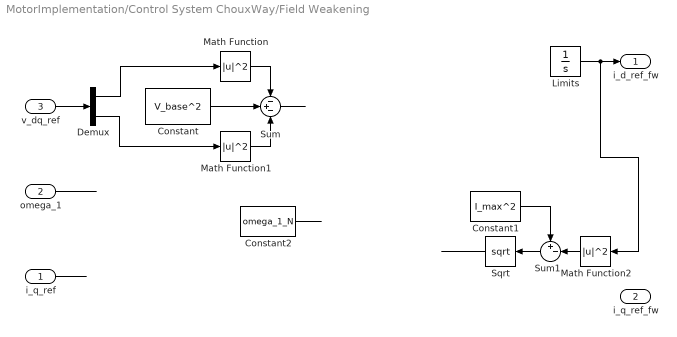
== system MotorImplementation/Control System ChouxWay/Field Weakening ==
  i_q_ref : Inport
  omega_1 : Inport  Port=2
  v_dq_ref : Inport  Port=3
  Constant : Constant  Value=V_base^2
  Constant1 : Constant  Value=I_max^2
  Constant2 : Constant  Value=omega_1_N
  Demux : Demux  Outputs=2
  Limits : Integrator  LimitOutput=on  UpperSaturationLimit=psi_ref/L_M_hat  LowerSaturationLimit=0.1*psi_ref/L_M_hat
  Math Function : Math  Operator=magnitude^2
  Math Function1 : Math  Operator=magnitude^2
  Math Function2 : Math  Operator=magnitude^2
  Sqrt : Sqrt
  Sum : Sum  Inputs=-+-
  Sum1 : Sum  Inputs=+-|
  i_d_ref_fw : Outport
  i_q_ref_fw : Outport  Port=2
  wires:
  Sum/1 -> ?
  ? -> i_q_ref_fw/1
  Constant2/1 -> ?
  ? -> Limits/1
  omega_1/1 -> ?
  Sqrt/1 -> ?
  v_dq_ref/1 -> Demux/1
  i_q_ref/1 -> ?
  Demux/2 -> Math Function1/1
  Constant1/1 -> Sum1/1
  Math Function1/1 -> Sum/3
  Demux/1 -> Math Function/1
  Sum1/1 -> Sqrt/1
  Math Function2/1 -> Sum1/2
  Constant/1 -> Sum/2
  Math Function/1 -> Sum/1
  Limits/1 -> Math Function2/1, i_d_ref_fw/1

== system MotorImplementation/Control System ChouxWay/FluxEstimator ==
  note: Initial condition: psi_ref
  i_dq_ref : Inport
  w_r : Inport  Port=2
  Demux1 : Demux  Outputs=2
  Gain : Gain  Gain=1/L_M_hat
  Gain1 : Gain  Gain=R_R_hat
  Gain2 : Gain  Gain=R_R_hat
  Integrator : Integrator  InitialCondition=psi_ref
  Product : Product  Inputs=/*
  Sum : Sum  Inputs=|+-
  Sum1 : Sum  Inputs=|++
  w_1 : Outport
  wires:
  Gain/1 -> Sum/2
  Sum/1 -> Gain1/1
  Demux1/1 -> Sum/1
  w_r/1 -> Sum1/2
  Integrator/1 -> Gain/1, Product/1
  Gain2/1 -> Sum1/1
  Product/1 -> Gain2/1
  Gain1/1 -> Integrator/1
  Demux1/2 -> Product/2
  Sum1/1 -> w_1/1
  i_dq_ref/1 -> Demux1/1

== system MotorImplementation/Control System ChouxWay/IM Motor ==
  In1 : Inport
  Out1 : Outport
  wires:
  In1/1 -> Out1/1

== system MotorImplementation/Control System ChouxWay/abc > dq ==
  In1 : Inport
  Out1 : Outport
  wires:
  In1/1 -> Out1/1

== system MotorImplementation/Control System ChouxWay/dq -> ABC ==
  In1 : Inport
  Out1 : Outport
  wires:
  In1/1 -> Out1/1

== system MotorImplementation/DrawWork/Bouyancy Force Comp ==
  Constant : Constant  Value=rho
  Display : Display
  Payload Volume : Constant  Value=Volume_pl
  Product : Product  Inputs=3
  gravity : Constant  Value=g
  B_force : Outport
  wires:
  Constant/1 -> Product/1
  Payload Volume/1 -> Product/2
  gravity/1 -> Product/3
  Product/1 -> Display/1, B_force/1

== system MotorImplementation/DrawWork/Subsystem ==
  Velocity : Inport
  MATLAB Function : MATLAB Function  TreatAsAtomicUnit=on
  F_Drag : Outport
  wires:
  Velocity/1 -> MATLAB Function/1(v)
  MATLAB Function/1(F_D) -> F_Drag/1

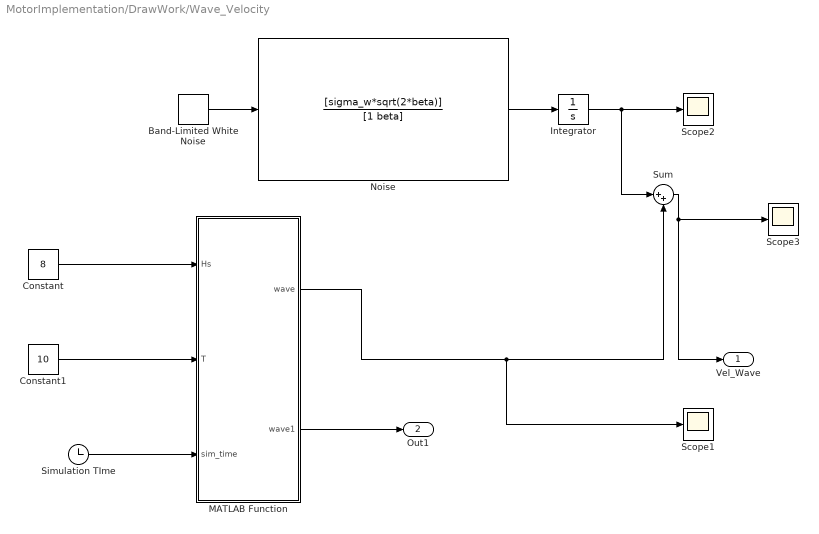
== system MotorImplementation/DrawWork/Wave_Velocity ==
  Band-Limited White Noise : simulink/Sources/Band-Limited White Noise  Cov=[1]  Ts=1/25  seed=[23341]
  Constant : Constant  Value=8
  Constant1 : Constant  Value=10
  Integrator : Integrator
  MATLAB Function : MATLAB Function  TreatAsAtomicUnit=on
  Noise : TransferFcn  Numerator=[sigma_w*sqrt(2*beta)]  Denominator=[1 beta]
  Scope1 : Scope
  Scope2 : Scope
  Scope3 : Scope
  Simulation TIme : Clock
      settings: Decimation=100
  Sum : Sum  Inputs=|++
  Vel_Wave : Outport
  Out1 : Outport  Port=2
  wires:
  Constant/1 -> MATLAB Function/1(Hs)
  Simulation TIme/1 -> MATLAB Function/3(sim_time)
  Constant1/1 -> MATLAB Function/2(T)
  MATLAB Function/1(wave) -> Sum/2, Scope1/1
  Band-Limited White Noise/1 -> Noise/1
  Noise/1 -> Integrator/1
  Sum/1 -> Vel_Wave/1, Scope3/1
  MATLAB Function/2(wave1) -> Out1/1
  Integrator/1 -> Sum/1, Scope2/1

== system MotorImplementation/FOC/Current Controller ==
  i_s_ref_dq : Inport
  v_sat_dq : Inport  Port=2
  i_s_dq : Inport  Port=3
  w_1 : Inport  Port=4
  MATLAB Function : MATLAB Function  TreatAsAtomicUnit=on
  Unit Delay : UnitDelay  SampleTime=-1  HasFrameUpgradeWarning=on
  v_s_ref_dq : Outport  PortDimensions=2
  wires:
  MATLAB Function/2(Inew) -> Unit Delay/1
  i_s_ref_dq/1 -> MATLAB Function/2(i_s_ref)
  w_1/1 -> MATLAB Function/4(w_1)
  i_s_dq/1 -> MATLAB Function/3(i_s)
  Unit Delay/1 -> MATLAB Function/5(I)
  MATLAB Function/1(v_s_ref) -> v_s_ref_dq/1
  v_sat_dq/1 -> MATLAB Function/1(v_sat_dq)

== system MotorImplementation/FOC/Field Weakening ==
  i_q_ref : Inport
  omega_1 : Inport  Port=2
  v_dq_ref : Inport  Port=3
  Constant : Constant  Value=0
  Demux : Demux  Outputs=2
  Magnitude Squared : Math  Operator=magnitude^2
  Magnitude Squared1 : Math  Operator=magnitude^2
  Sum : Sum  Inputs=-+-
  i_q_ref_fw : Outport
  i_d_ref_fw : Outport  Port=2
  wires:
  v_dq_ref/1 -> Demux/1
  Demux/2 -> Magnitude Squared1/1
  Demux/1 -> Magnitude Squared/1
  Magnitude Squared/1 -> Sum/1
  Magnitude Squared1/1 -> Sum/3
  Constant/1 -> Sum/2

== system MotorImplementation/FOC/Flux Estimation ==
  i_d_ref.fw : Inport
  i_q_ref.fw : Inport  Port=2
  omega_actual : Inport  Port=3
  Add : Sum
  Divide : Product  Inputs=/*
  Gain : Gain  Gain=RR_Hat
  Gain1 : Gain  Gain=RR_Hat
  Gain2 : Gain  Gain=1/L_M_hat
  Integrator : Integrator
  Sum : Sum  Inputs=|+-
  omega_1 : Outport
  wires:
  i_d_ref.fw/1 -> Sum/1
  Sum/1 -> Gain/1
  Gain/1 -> Integrator/1
  Divide/1 -> Gain1/1
  Gain1/1 -> Add/1
  Add/1 -> omega_1/1
  Integrator/1 -> Gain2/1, Divide/1
  Gain2/1 -> Sum/2
  i_q_ref.fw/1 -> Divide/2
  omega_actual/1 -> Add/2

== system MotorImplementation/FOC/IM-Model ==
  vs_abc : Inport
  w_m : Inport  Port=2
  Electromagnetic Torque : Subsystem
  Flux Equations : Subsystem
  Gain : Gain  Gain=n_p  SaturateOnIntegerOverflow=on  OutDataTypeStr=Inherit: Same as input  ParamDataTypeStr=Inherit: Same as input
  Voltage Equations : Subsystem
  abc->alphabeta : Subsystem
  alphabeta->abc : Subsystem
  is_abc : Outport
  T_em : Outport  Port=2
  wires:
  Flux Equations/2(i_R^s) -> Voltage Equations/4(i_R^s)
  Electromagnetic Torque/1(T_em) -> T_em/1
  Flux Equations/1(i_s^s) -> Electromagnetic Torque/1(i_s^s), Voltage Equations/2(i_s^s), alphabeta->abc/1(i_s^s)
  w_m/1 -> Gain/1
  Gain/1 -> Voltage Equations/3(w_r)
  alphabeta->abc/1(is_abc) -> is_abc/1
  vs_abc/1 -> abc->alphabeta/1(vs_abc)
  Voltage Equations/2(psi_R^s) -> Flux Equations/2(psi_R^s), Electromagnetic Torque/2(psi_R^s)
  abc->alphabeta/1(v_s^s) -> Voltage Equations/1(v_s^s)
  Voltage Equations/1(psi_s^s) -> Flux Equations/1(psi_s^s)

== system MotorImplementation/FOC/abc->dq1 ==
  is_abc : Inport
  thetas : Inport  Port=2
  MATLAB Function : MATLAB Function  TreatAsAtomicUnit=on
  is_dq : Outport
  wires:
  MATLAB Function/1(is) -> is_dq/1
  thetas/1 -> MATLAB Function/2(thetas)
  is_abc/1 -> MATLAB Function/1(is_abc)

== system MotorImplementation/FOC/dq->abc ==
  vs_dq : Inport
  thetas : Inport  Port=2
  MATLAB Function : MATLAB Function  TreatAsAtomicUnit=on
  vs_abc : Outport
  wires:
  MATLAB Function/1(vs_abc) -> vs_abc/1
  thetas/1 -> MATLAB Function/2(thetas)
  vs_dq/1 -> MATLAB Function/1(vs_dq)

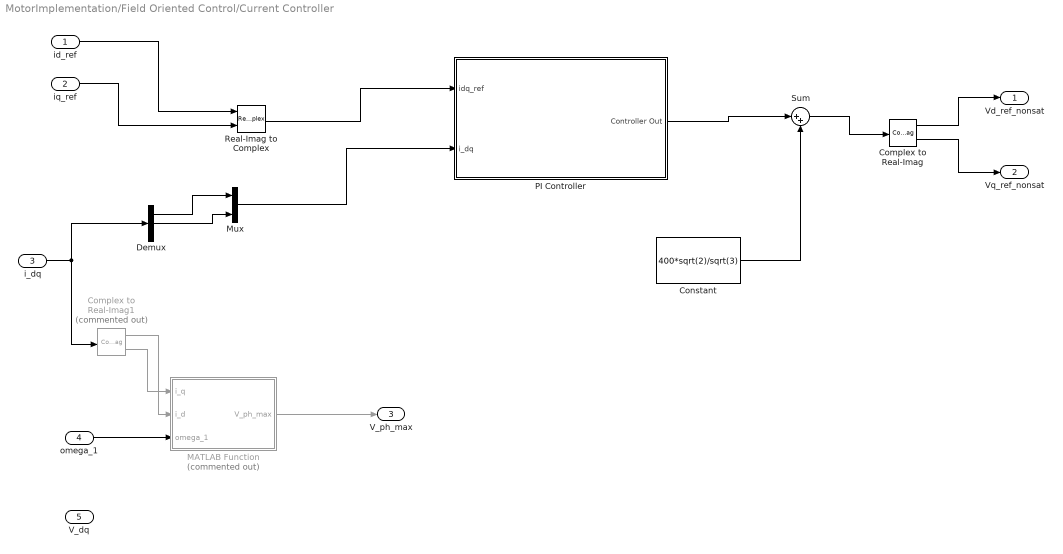
== system MotorImplementation/Field Oriented Control/Current Controller ==
  id_ref : Inport
  iq_ref : Inport  Port=2
  i_dq : Inport  Port=3
  omega_1 : Inport  Port=4
  V_dq : Inport  Port=5
  Complex to Real-Imag : ComplexToRealImag
  Complex to Real-Imag1 : ComplexToRealImag  Commented=on
  Constant : Constant  Value=400*sqrt(2)/sqrt(3)
  Demux : Demux  Outputs=3
  MATLAB Function : MATLAB Function  Commented=on  TreatAsAtomicUnit=on
  Mux : Mux  Inputs=2
  PI Controller : Subsystem
  Real-Imag to Complex : RealImagToComplex
  Sum : Sum  Inputs=|++
  Vd_ref_nonsat : Outport
  Vq_ref_nonsat : Outport  Port=2
  V_ph_max : Outport  Port=3
  wires:
  i_dq/1 -> Complex to Real-Imag1/1, Demux/1
  Complex to Real-Imag1/1 -> MATLAB Function/2(i_d)
  Complex to Real-Imag1/2 -> MATLAB Function/1(i_q)
  omega_1/1 -> MATLAB Function/3(omega_1)
  id_ref/1 -> Real-Imag to Complex/1
  iq_ref/1 -> Real-Imag to Complex/2
  Real-Imag to Complex/1 -> PI Controller/1(idq_ref)
  PI Controller/1(Controller Out) -> Sum/1
  Sum/1 -> Complex to Real-Imag/1
  Complex to Real-Imag/1 -> Vd_ref_nonsat/1
  Complex to Real-Imag/2 -> Vq_ref_nonsat/1
  MATLAB Function/1(V_ph_max) -> V_ph_max/1
  Demux/1 -> Mux/1
  Demux/2 -> Mux/2
  Mux/1 -> PI Controller/2(i_dq)
  Constant/1 -> Sum/2

== system MotorImplementation/Field Oriented Control/Flux Controller ==
  I_magnetizing_rotor : Inport
  i_mr_ref : Inport  Port=2
  Complex to Real-Imag1 : ComplexToRealImag
  Constant : Constant  Value=185
  PID Controller : slpidlib/PID Controller  Controller=PI  Form=Parallel  TimeDomain=Discrete-time  UseExternalTs=off  SampleTime=-1  IntegratorMethod=Forward Euler  FilterMethod=Forward Euler  ControllerParametersSource=internal  P=100  I=3000  UseKiTs=off  D=0  N=100  UseFilter=on  TunerSelectOption=Transfer Function Based (PID Tuner App)  InitialConditionSource=internal  InitialConditionForIntegrator=0  InitialConditionForFilter=0  DifferentiatorICPrevScaledInput=0  ExternalReset=none  TrackingMode=off  Kt=1  LimitOutput=off  SatLimitsSource=internal  UpperSaturationLimit=inf  LowerSaturationLimit=-inf  LinearizeAsGain=on  AntiWindupMode=none  Kb=1  POutMin=[]  POutMax=[]  IOutMin=[]  IOutMax=[]  DOutMin=[]  DOutMax=[]  NOutMin=[]  NOutMax=[]  SumOutMin=[]  SumOutMax=[]  SaturationOutMin=[]  SaturationOutMax=[]  PParamMin=[]  PParamMax=[]  IParamMin=[]  IParamMax=[]  DParamMin=[]  DParamMax=[]  NParamMin=[]  NParamMax=[]  KbParamMin=[]  KbParamMax=[]  KtParamMin=[]  KtParamMax=[]  KbOutMin=[]  KbOutMax=[]  KtOutMin=[]  KtOutMax=[]  IntegratorOutMin=[]  IntegratorOutMax=[]  FilterOutMin=[]  FilterOutMax=[]  SumI1OutMin=[]  SumI1OutMax=[]  SumI2OutMin=[]  SumI2OutMax=[]  SumI3OutMin=[]  SumI3OutMax=[]  SumI4OutMin=[]  SumI4OutMax=[]  SumDOutMin=[]  SumDOutMax=[]  DifferentiatorOutMin=[]  DifferentiatorOutMax=[]  FilterDiffOutCoefMin=[]  FilterDiffOutCoefMax=[]  ReciprocalOutMin=[]  ReciprocalOutMax=[]  SumDenOutMin=[]  SumDenOutMax=[]  SumNumOutMin=[]  SumNumOutMax=[]  DivideOutMin=[]  DivideOutMax=[]  UdiffTsProdOutMin=[]  UdiffTsProdOutMax=[]  NTsProdOutMin=[]  NTsProdOutMax=[]  UintegralTsProdOutMin=[]  UintegralTsProdOutMax=[]  UngainTsProdOutMin=[]  UngainTsProdOutMax=[]  IntegratorContinuousStateAttributes=''  IntegratorStateMustResolveToSignalObject=off  IntegratorRTWStateStorageClass=Auto  FilterContinuousStateAttributes=''  FilterStateMustResolveToSignalObject=off  FilterRTWStateStorageClass=Auto  ParallelPVariant=InternalParameters  IdealPVariant=Disabled  IVariant=InternalParameters  DVariant=Disabled  IntegratorVariant=Discrete  SatVariant=Disabled  AWVariant=Passthrough  PCopyVariant=Disabled  TRVariant=Disabled  FdbkBlocksVariant=Forward  IdealPFdbkVariant=Disabled  SatFdbkVariant=Disabled  DerivativeFilterVariant=Disabled  NVariant=Disabled  NCopyVariant=Disabled_SignalSpec  FilterICVariant=Disabled  IntegratorICVariant=InternalICs  ExternalResetVariant=Disabled  TRSumVariant=Passthrough  SumFdbkVariant=Disabled  SumVariant=Sum_PI  TsampFilterVariant=InternalTs  TsampNgainVariant=Passthrough  TsampIntegralVariant=Passthrough  ExternalSaturationOutDataTypeStr=Inherit: Same as second input  aMode=0
  Scope : Scope
  Sum : Sum  Inputs=|+-
  id_ref : Outport
  wires:
  PID Controller/1 -> id_ref/1
  i_mr_ref/1 -> ?
  Constant/1 -> Sum/1
  I_magnetizing_rotor/1 -> Sum/2, Complex to Real-Imag1/1
  Sum/1 -> Scope/1, PID Controller/1

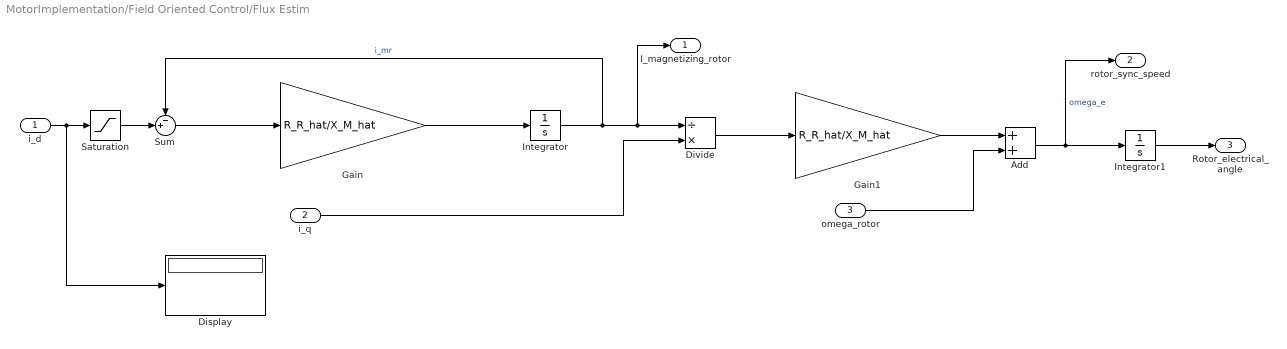
== system MotorImplementation/Field Oriented Control/Flux Estim ==
  i_d : Inport
  i_q : Inport  Port=2
  omega_rotor : Inport  Port=3
  Add : Sum
  Display : Display
  Divide : Product  Inputs=/*
  Gain : Gain  Gain=R_R_hat/X_M_hat
  Gain1 : Gain  Gain=R_R_hat/X_M_hat
  Integrator : Integrator  InitialCondition=psi_R
  Integrator1 : Integrator
  Saturation : Saturate  UpperLimit=200  LowerLimit=0.001
  Sum : Sum  Inputs=-+|
  I_magnetizing_rotor : Outport
  rotor_sync_speed : Outport  Port=2
  Rotor_electrical_angle : Outport  Port=3
  wires:
  Gain/1 -> Integrator/1
  Integrator/1 -> I_magnetizing_rotor/1, Divide/1, Sum/1  "i_mr"
  i_q/1 -> Divide/2
  Divide/1 -> Gain1/1
  Gain1/1 -> Add/1
  omega_rotor/1 -> Add/2
  Add/1 -> rotor_sync_speed/1, Integrator1/1  "omega_e"
  Integrator1/1 -> Rotor_electrical_angle/1
  Sum/1 -> Gain/1
  i_d/1 -> Display/1, Saturation/1
  Saturation/1 -> Sum/2

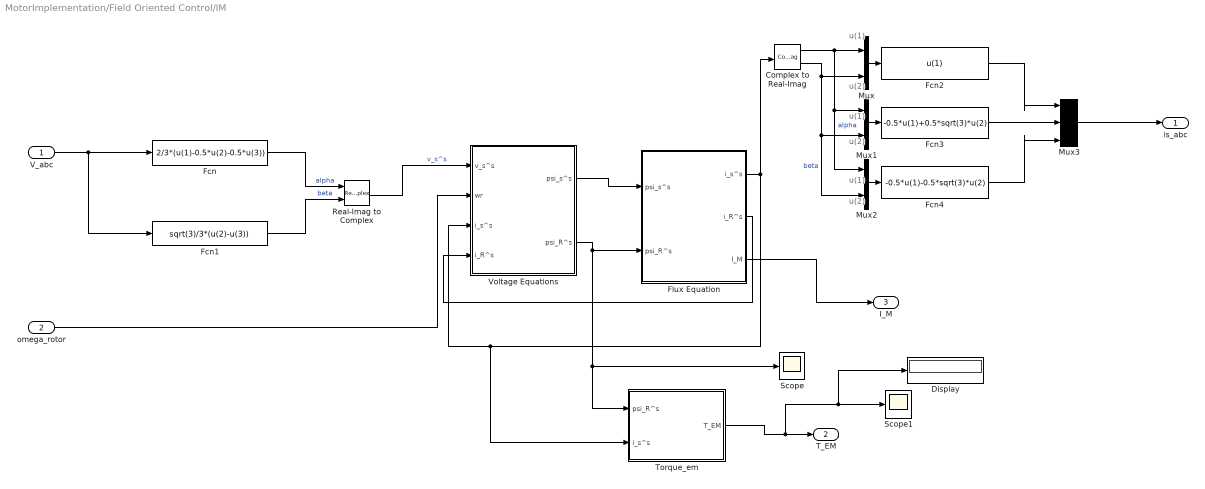
== system MotorImplementation/Field Oriented Control/IM ==
  note: u(1)
  note: u(2)
  note: u(2)
  note: u(2)
  note: u(1)
  note: u(1)
  V_abc : Inport
  omega_rotor : Inport  Port=2
  Complex to Real-Imag : ComplexToRealImag
  Display : Display
  Fcn : Fcn  Expr=2/3*(u(1)-0.5*u(2)-0.5*u(3))
  Fcn1 : Fcn  Expr=sqrt(3)/3*(u(2)-u(3))
  Fcn2 : Fcn  Expr=u(1)
  Fcn3 : Fcn  Expr=-0.5*u(1)+0.5*sqrt(3)*u(2)
  Fcn4 : Fcn  Expr=-0.5*u(1)-0.5*sqrt(3)*u(2)
  Flux Equation : Subsystem
  Mux : Mux  Inputs=2
  Mux1 : Mux  Inputs=2
  Mux2 : Mux  Inputs=2
  Mux3 : Mux  Inputs=3
  Real-Imag to Complex : RealImagToComplex
  Scope : Scope
  Scope1 : Scope
  Torque_em : Subsystem
  Voltage Equations : Subsystem
  is_abc : Outport
  T_EM : Outport  Port=2
  I_M : Outport  Port=3
  wires:
  V_abc/1 -> Fcn1/1, Fcn/1
  Fcn/1 -> Real-Imag to Complex/1  "alpha"
  Fcn1/1 -> Real-Imag to Complex/2  "beta"
  Real-Imag to Complex/1 -> Voltage Equations/1(v_s^s)  "v_s^s"
  omega_rotor/1 -> Voltage Equations/2(wr)
  Voltage Equations/1(psi_s^s) -> Flux Equation/1(psi_s^s)
  Voltage Equations/2(psi_R^s) -> Scope/1, Torque_em/1(psi_R^s), Flux Equation/2(psi_R^s)
  Complex to Real-Imag/1 -> Mux2/1, Mux1/1, Mux/1  "alpha"
  Mux/1 -> Fcn2/1
  Complex to Real-Imag/2 -> Mux2/2, Mux1/2, Mux/2  "beta"
  Mux2/1 -> Fcn4/1
  Flux Equation/1(i_s^s) -> Torque_em/2(i_s^s), Voltage Equations/3(i_s^s), Complex to Real-Imag/1
  Mux1/1 -> Fcn3/1
  Fcn4/1 -> Mux3/3
  Fcn3/1 -> Mux3/2
  Fcn2/1 -> Mux3/1
  Mux3/1 -> is_abc/1
  Flux Equation/2(i_R^s) -> Voltage Equations/4(i_R^s)
  Torque_em/1(T_EM) -> Display/1, Scope1/1, T_EM/1
  Flux Equation/3(I_M) -> I_M/1

== system MotorImplementation/Field Oriented Control/Saturation ==
  Vd_ref_nonsat : Inport
  Vq_ref_nonsat : Inport  Port=2
  V_ph_max : Inport  Port=3
  Complex to Magnitude-Angle : ComplexToMagnitudeAngle
  Complex to Real-Imag : ComplexToRealImag
  Magnitude-Angle to Complex : MagnitudeAngleToComplex
  Mux : Mux  Inputs=2
  Real-Imag to Complex : RealImagToComplex
  Saturation : Saturate  UpperLimit=400/sqrt(3) * sqrt(2)  LowerLimit=0
  v_dq_sat : Outport
  wires:
  Vd_ref_nonsat/1 -> Real-Imag to Complex/1
  Vq_ref_nonsat/1 -> Real-Imag to Complex/2
  Real-Imag to Complex/1 -> Complex to Magnitude-Angle/1
  Complex to Magnitude-Angle/1 -> Saturation/1
  Saturation/1 -> Magnitude-Angle to Complex/1
  Complex to Magnitude-Angle/2 -> Magnitude-Angle to Complex/2
  Magnitude-Angle to Complex/1 -> Complex to Real-Imag/1
  Complex to Real-Imag/1 -> Mux/1
  Complex to Real-Imag/2 -> Mux/2
  Mux/1 -> v_dq_sat/1
